simulink model "Autopilot_pwa_mdl"  (R2018b)
settings: Solver=VariableStepAuto  StartTime=0.0  StopTime=3  MaxStep=0.01  RelTol=1e-3
libraries: cstblocks x3, lpvlibrary x2, simulink x1
settings Model: Creator=ferna  LastModifiedBy=ferna

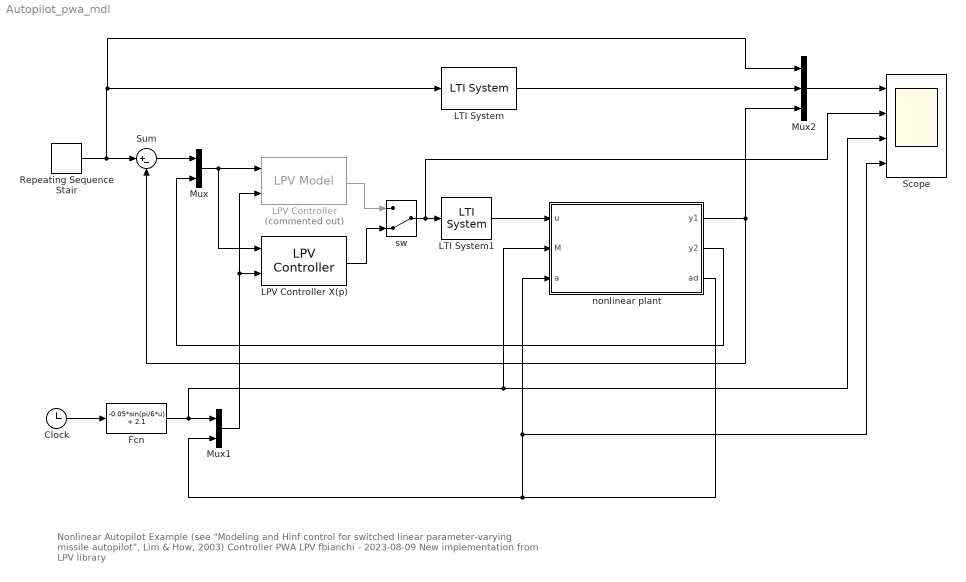
== system Autopilot_pwa_mdl ==
  note: Nonlinear Autopilot Example (see "Modeling and Hinf control for switched linear parameter-varying missile autopilot", Lim & How, 2003)
      | Controller PWA LPV
      | fbianchi - 2023-08-09
      | New implementation from LPV library
  Clock : Clock
  Fcn : Fcn  Expr=-0.05*sin(pi/6*u) + 2.1
  LPV Controller : lpvlibrary/LPV Model  Commented=on  pdG=pdK  x0=0
      settings: SourceProductName=LPV Toolbox
  LPV Controller X(p) : lpvlibrary/LPV Controller  pdK=pdK  x0=0
      settings: SourceProductName=LPV Toolbox
  LTI System : cstblocks/LTI System  sys=Wref  IC=[]
  LTI System1 : cstblocks/LTI System  sys=Act  IC=[]
  Mux : Mux  Inputs=2
  Mux1 : Mux  Inputs=2
  Mux2 : Mux  Inputs=3
  Repeating Sequence Stair : simulink/Sources/Repeating Sequence Stair  OutValues=[10 -15 0 0].'  tsamp=1  OutMin=[]  OutMax=[]  OutDataTypeStr=double  OutputDataTypeScalingMode=double  OutDataType=fixdt(0,8)  ConRadixGroup=Best Precision: Vector-wise  OutScaling=2^-12
  Scope : Scope  NumInputPorts=4
  Sum : Sum  Inputs=|+-
  nonlinear plant : Subsystem
  sw : ManualSwitch  CurrentSetting=0
  wires:
  LTI System1/1 -> nonlinear plant/1(u)
  Mux/1 -> LPV Controller/1, LPV Controller X(p)/1
  Sum/1 -> Mux/1
  nonlinear plant/2(y2) -> Mux/2
  nonlinear plant/1(y1) -> Mux2/3, Sum/2
  Clock/1 -> Fcn/1
  Fcn/1 -> nonlinear plant/2(M), Scope/3, Mux1/1
  Mux1/1 -> LPV Controller/2, LPV Controller X(p)/2
  Repeating Sequence Stair/1 -> LTI System/1, Mux2/1, Sum/1
  Mux2/1 -> Scope/1
  LTI System/1 -> Mux2/2
  nonlinear plant/3(ad) -> Mux1/2, nonlinear plant/3(a), Scope/4
  LPV Controller/1 -> sw/1
  sw/1 -> Scope/2, LTI System1/1
  LPV Controller X(p)/1 -> sw/2

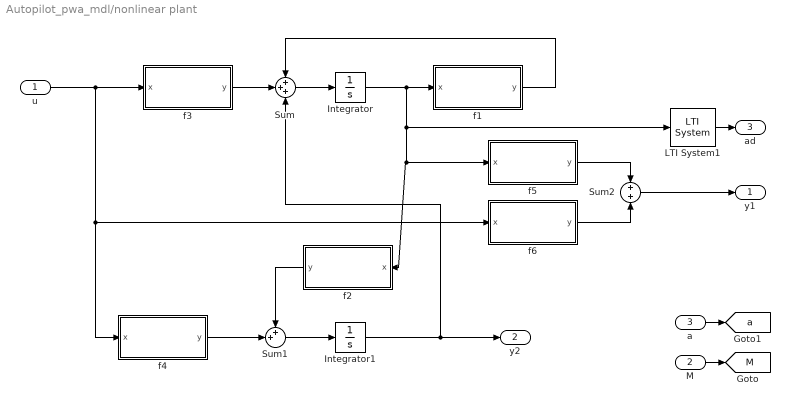
== system Autopilot_pwa_mdl/nonlinear plant ==
  u : Inport
  M : Inport  Port=2
  a : Inport  Port=3
  Integrator : Integrator
  Integrator1 : Integrator
  LTI System1 : cstblocks/LTI System  sys=F  IC=[]
  Sum : Sum  Inputs=+++
  Sum1 : Sum  Inputs=++|
  Sum2 : Sum
  f1 : Subsystem
  f2 : Subsystem
  f3 : Subsystem
  f4 : Subsystem
  f5 : Subsystem
  f6 : Subsystem
  y1 : Outport
  y2 : Outport  Port=2
  ad : Outport  Port=3
  tag scope: M=global, a=global
  wires:
  a/1 -> [a]
  f6/1(y) -> Sum2/2
  M/1 -> [M]
  f1/1(y) -> Sum/1
  f3/1(y) -> Sum/2
  Integrator/1 -> f2/1(x), f5/1(x), LTI System1/1, f1/1(x)
  Integrator1/1 -> Sum/3, y2/1
  f5/1(y) -> Sum2/1
  Sum/1 -> Integrator/1
  u/1 -> f6/1(x), f4/1(x), f3/1(x)
  Sum2/1 -> y1/1
  LTI System1/1 -> ad/1
  Sum1/1 -> Integrator1/1
  f4/1(y) -> Sum1/2
  f2/1(y) -> Sum1/1

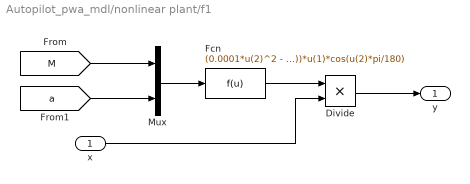
== system Autopilot_pwa_mdl/nonlinear plant/f1 ==
  x : Inport
  Divide : Product  Inputs=**
  Fcn : Fcn  Expr=(0.0001*u(2)^2 - 0.0112*abs(u(2)) - 0.2010*(2 - u(1)/3))*u(1)*cos(u(2)*pi/180)
  Mux : Mux  Inputs=2
  y : Outport
  wires:
  [a] -> Mux/2
  Mux/1 -> Fcn/1
  [M] -> Mux/1
  Fcn/1 -> Divide/1
  Divide/1 -> y/1
  x/1 -> Divide/2

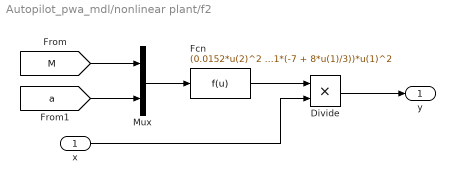
== system Autopilot_pwa_mdl/nonlinear plant/f2 ==
  x : Inport
  Divide : Product  Inputs=**
  Fcn : Fcn  Expr=(0.0152*u(2)^2 - 1.3765*abs(u(2)) + 3.6001*(-7 + 8*u(1)/3))*u(1)^2
  Mux : Mux  Inputs=2
  y : Outport
  wires:
  x/1 -> Divide/2
  Divide/1 -> y/1
  Fcn/1 -> Divide/1
  [M] -> Mux/1
  Mux/1 -> Fcn/1
  [a] -> Mux/2

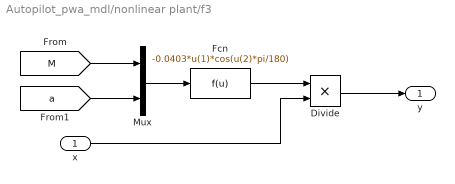
== system Autopilot_pwa_mdl/nonlinear plant/f3 ==
  x : Inport
  Divide : Product  Inputs=**
  Fcn : Fcn  Expr=-0.0403*u(1)*cos(u(2)*pi/180)
  Mux : Mux  Inputs=2
  y : Outport
  wires:
  Mux/1 -> Fcn/1
  Fcn/1 -> Divide/1
  Divide/1 -> y/1
  x/1 -> Divide/2
  [a] -> Mux/2
  [M] -> Mux/1

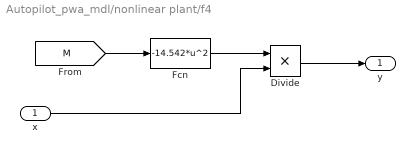
== system Autopilot_pwa_mdl/nonlinear plant/f4 ==
  x : Inport
  Divide : Product  Inputs=**
  Fcn : Fcn  Expr=-14.542*u^2
  y : Outport
  wires:
  x/1 -> Divide/2
  Divide/1 -> y/1
  Fcn/1 -> Divide/1
  [M] -> Fcn/1

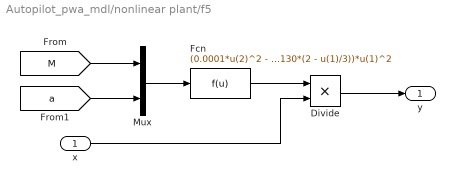
== system Autopilot_pwa_mdl/nonlinear plant/f5 ==
  x : Inport
  Divide : Product  Inputs=**
  Fcn : Fcn  Expr=(0.0001*u(2)^2 - 0.0063*abs(u(2)) - 0.1130*(2 - u(1)/3))*u(1)^2
  Mux : Mux  Inputs=2
  y : Outport
  wires:
  Mux/1 -> Fcn/1
  Fcn/1 -> Divide/1
  Divide/1 -> y/1
  x/1 -> Divide/2
  [a] -> Mux/2
  [M] -> Mux/1

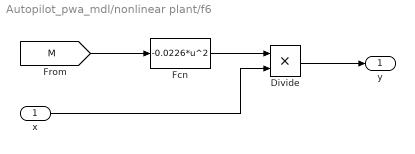
== system Autopilot_pwa_mdl/nonlinear plant/f6 ==
  x : Inport
  Divide : Product  Inputs=**
  Fcn : Fcn  Expr=-0.0226*u^2
  y : Outport
  wires:
  x/1 -> Divide/2
  Divide/1 -> y/1
  Fcn/1 -> Divide/1
  [M] -> Fcn/1
